simulink model "primer01_2012"  (R2016b)
settings: Solver=VariableStepAuto  StartTime=0.0  StopTime=10.0  FixedStep=0.01  MaxStep=0.01  RelTol=1e-3  EnableMultiTasking=on
values from neighbouring files (symbols this model uses):
  T = 0.1    [Zadatak1_konstatnte.m]    (also in primer01_konstante.m = 1; primer06_konstante.m)
settings Model: Creator=Vukan  LastModifiedBy=User
settings SolverCC: InsertRTBMode=Never (minimum delay)
settings OptimizationCC: LifeSpan=inf
settings DebuggingCC: SFUnexpectedBacktrackingDiag=warning  SFNoUnconditionalDefaultTransitionDiag=warning  SFExecutionAtInitializationDiag=none
settings GRTTargetCC: TargetLangStandard=C89/C90 (ANSI)  GeneratePreprocessorConditionals=Disable all
settings ConfigComp: CovMetricSettings=dw  CovHtmlReporting=on  CovSaveCumulativeToWorkspaceVar=on  CovSaveSingleToWorkspaceVar=on  CovExternalEMLEnable=off

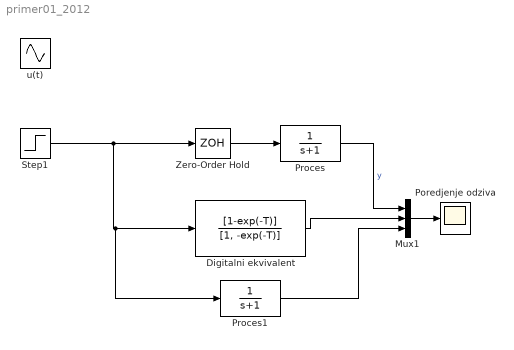
== system primer01_2012 ==
  Digitalni ekvivalent : DiscreteTransferFcn  Numerator=[1-exp(-T)]  Denominator=[1, -exp(-T)]  SampleTime=T
  Mux1 : Mux  Inputs=3
  Poredjenje odziva : Scope
  Proces : TransferFcn  Denominator=[1 1]
  Proces1 : TransferFcn  Denominator=[1 1]
  Step1 : Step  Time=0  SampleTime=0
  Zero-Order Hold : ZeroOrderHold  SampleTime=T
  u(t) : Sin  Frequency=0.5  SampleTime=0
  wires:
  Mux1/1 -> Poredjenje odziva/1
  Digitalni ekvivalent/1 -> Mux1/2
  Proces1/1 -> Mux1/3
  Proces/1 -> Mux1/1  "y"
  Zero-Order Hold/1 -> Proces/1
  Step1/1 -> Proces1/1, Digitalni ekvivalent/1, Zero-Order Hold/1
